simulink model "model_quad_nl_mpc_nl"  (R2021b)
settings: Solver=FixedStepAuto  StartTime=0.0  StopTime=10  FixedStep=.01  MaxStep=.1  MinStep=.005  RelTol=1e-3
values from neighbouring files (symbols this model uses):
  Abody = pi*Rbody^2    (= 0.0314159265359)    [model_quad_init.m]    (also in nlStateFcn.m = 0.0314)
  CDbody = 0.75    [model_quad_init.m]    (also in nlStateFcn.m)
  CT = 0.0248    [model_quad_init.m]
  g = 9.81    [model_quad_init.m]    (also in nlStateFcn.m; nlStateFcnTest.m; start_drone.m)
  i0 = 0    [model_quad_init.m]    (also in nlStateFcn.m)
  Ibbperp = .00942    (= 0.00942)    [model_quad_init.m]    (also in nlStateFcn.m; nlStateFcnTest.m)
  Ibbxx = Ibbperp    (= 0.00942)    [model_quad_init.m]    (also in nlStateFcn.m; nlStateFcnTest.m)
  Ibbxz = 0    [model_quad_init.m]    (also in nlStateFcn.m; nlStateFcnTest.m)
  Ibbyy = Ibbperp    (= 0.00942)    [model_quad_init.m]    (also in nlStateFcn.m; nlStateFcnTest.m)
  Ibbzz = .01867    (= 0.01867)    [model_quad_init.m]    (also in nlStateFcn.m; nlStateFcnTest.m)
  Irrperp = Irrpolar/2    (= 0.0001113)    [model_quad_init.m]    (also in nlStateFcn.m; nlStateFcnTest.m)
  Irrpolar = .0002226    (= 0.0002226)    [model_quad_init.m]
  Kv = 130    [model_quad_init.m]    (also in nlStateFcn.m)
  mb = mb/m_tot    (= 0.760306807287)    [model_quad_init.m]    (also in nlStateFcn.m; nlStateFcnTest.m)
  mr = mr/m_tot    (= 0.0599232981783)    [model_quad_init.m]    (also in nlStateFcn.m; nlStateFcnTest.m)
  R_arms = .45/2    (= 0.225)    [model_quad_init.m]    (also in nlStateFcn.m; nlStateFcnTest.m)
  R_rotor = .125    (= 0.125)    [model_quad_init.m]    (also in nlStateFcn.m)
  rho = 1.225    [model_quad_init.m]    (also in nlStateFcn.m)
  rotorAero = load('loopQuadBET_fromTheBook.mat','C_T','C_H','C_M','C_Q','mu_z_loops','mu_x_loops')    [model_quad_init.m]    (also in nlStateFcn.m)
  Rwinding = 0.56    [model_quad_init.m]
  spin_dir = [1 -1 1 -1]    [model_quad_init.m]    (also in nlStateFcn.m = [1,-1,1,-1])
  Vmax = 4*3.7    (= 14.8)    [model_quad_init.m]
  z_rotors = 0    [model_quad_init.m]    (also in nlStateFcn.m; nlStateFcnTest.m)
undefined symbols (not defined in the file or in its folder): R_RB
libraries: dspmathops x1, mpclib x1
(part 2 of 2)

== matlab function model_quad_nl_mpc_nl/NL Drone Model/Aerodynamics/rotor aerodynamics2/MATLAB Function ==
  data: Omega1 input; Omega2 input; Omega3 input; Omega4 input; R input; phi input; psi input; theta input; u input; mu output; v input; w input; w_xE input; w_yE input; w_zE input
function mu = ODE_quad_advanceratios(Omega1,Omega2,Omega3,Omega4,R,phi,psi,theta,u,v,w,w_xE,w_yE,w_zE)
%ODE_QUAD_ADVANCERATIOS
%    MU = ODE_QUAD_ADVANCERATIOS(OMEGA1,OMEGA2,OMEGA3,OMEGA4,R,PHI,PSI,THETA,U,V,W,W_XE,W_YE,W_ZE)

%    This function was generated by the Symbolic Math Toolbox version 8.5.
%    12-Apr-2021 01:36:09

t2 = cos(phi);
t3 = cos(psi);
t4 = cos(theta);
t5 = sin(phi);
t6 = sin(psi);
t7 = sin(theta);
t8 = 1.0./Omega1;
t9 = 1.0./Omega2;
t10 = 1.0./Omega3;
t11 = 1.0./Omega4;
t12 = 1.0./R;
t13 = t7.*w_zE;
t14 = t2.*t3;
t15 = t2.*t6;
t16 = t3.*t5;
t17 = t5.*t6;
t18 = t2.*t4.*w_zE;
t19 = t3.*t4.*w_xE;
t20 = t4.*t5.*w_zE;
t21 = t4.*t6.*w_yE;
t22 = t7.*t17;
t23 = t7.*t14;
t24 = t7.*t15;
t25 = t7.*t16;
t26 = -t18;
t27 = -t19;
t28 = -t20;
t29 = -t21;
t30 = -t24;
t31 = -t25;
t32 = t14+t22;
t33 = t17+t23;
t42 = t13+t27+t29+u;
t34 = t33.*w_xE;
t35 = t32.*w_yE;
t36 = t15+t31;
t37 = t16+t30;
t43 = t42.^2;
t38 = t36.*w_xE;
t39 = -t34;
t40 = t37.*w_yE;
t41 = -t35;
t44 = t28+t38+t41+v;
t45 = t26+t39+t40+w;
t46 = (t20+t35-t38-v).^2;
t47 = t43+t46;
t48 = 1.0./sqrt(t47);
t49 = t43.*t48;
t50 = t46.*t48;
t51 = t49+t50;
mu = [t8.*t12.*(t18+t34-t40-w);-t8.*t12.*t51;t9.*t12.*(t18+t34-t40-w);-t9.*t12.*t51;t10.*t12.*(t18+t34-t40-w);-t10.*t12.*t51;t11.*t12.*(t18+t34-t40-w);-t11.*t12.*t51];

== matlab function model_quad_nl_mpc_nl/NL Drone Model/Aerodynamics/rotor aerodynamics2/MATLAB Function1 ==
  data: CH1 input; CH2 input; CH3 input; CH4 input; CM1 input; FR output; CM2 input; CM3 input; CM4 input; CQ1 input; CQ2 input; CQ3 input; CQ4 input; CT1 input; CT2 input; CT3 input; CT4 input; Omega1 input; Omega2 input; Omega3 input; Omega4 input; R input; phi input; theta input; psi input; rho input; u input; v input; w_xE input; w_yE input; w_zE input
function FR = ODE_quad_rotorforces(CH1,CH2,CH3,CH4,CM1,CM2,CM3,CM4,CQ1,CQ2,CQ3,CQ4,CT1,CT2,CT3,CT4,Omega1,Omega2,Omega3,Omega4,R,phi,theta,psi,rho,u,v,w_xE,w_yE,w_zE)
%ODE_QUAD_ROTORFORCES
%    FR = ODE_QUAD_ROTORFORCES(CH1,CH2,CH3,CH4,CM1,CM2,CM3,CM4,CQ1,CQ2,CQ3,CQ4,CT1,CT2,CT3,CT4,OMEGA1,OMEGA2,OMEGA3,OMEGA4,R,PHI,PSI,RHO,THETA,U,V,W_XE,W_YE,W_ZE)

%    This function was generated by the Symbolic Math Toolbox version 8.5.
%    12-Apr-2021 00:26:00

t2 = cos(phi);
t3 = cos(psi);
t4 = cos(theta);
t5 = sin(phi);
t6 = sin(psi);
t7 = sin(theta);
t8 = Omega1.^2;
t9 = Omega2.^2;
t10 = Omega3.^2;
t11 = Omega4.^2;
t12 = R.^4;
t13 = R.^5;
t14 = t7.*w_zE;
t15 = t2.*t3;
t16 = t2.*t6;
t17 = t3.*t4.*w_xE;
t18 = t4.*t5.*w_zE;
t19 = t4.*t6.*w_yE;
t20 = t5.*t6.*t7;
t21 = t3.*t5.*t7;
t22 = -t17;
t23 = -t18;
t24 = -t19;
t25 = -t21;
t26 = t15+t20;
t27 = t26.*w_yE;
t28 = t16+t25;
t31 = t14+t22+t24+u;
t29 = t28.*w_xE;
t30 = -t27;
t32 = t31.^2;
t33 = t23+t29+t30+v;
t34 = (t18+t27-t29-v).^2;
t35 = t32+t34;
t36 = 1.0./sqrt(t35);
FR = [CH1.*rho.*t8.*t12.*t31.*t36.*pi.*(-1.0./2.0);CH2.*rho.*t9.*t12.*t31.*t36.*pi.*(-1.0./2.0);CH3.*rho.*t10.*t12.*t31.*t36.*pi.*(-1.0./2.0);CH4.*rho.*t11.*t12.*t31.*t36.*pi.*(-1.0./2.0);CH1.*rho.*t8.*t12.*t36.*pi.*(t18+t27-t29-v).*(-1.0./2.0);CH2.*rho.*t9.*t12.*t36.*pi.*(t18+t27-t29-v).*(-1.0./2.0);CH3.*rho.*t10.*t12.*t36.*pi.*(t18+t27-t29-v).*(-1.0./2.0);CH4.*rho.*t11.*t12.*t36.*pi.*(t18+t27-t29-v).*(-1.0./2.0);(CT1.*rho.*t8.*t12.*pi)./2.0;(CT2.*rho.*t9.*t12.*pi)./2.0;(CT3.*rho.*t10.*t12.*pi)./2.0;(CT4.*rho.*t11.*t12.*pi)./2.0;(CM1.*rho.*t8.*t13.*t31.*t36.*pi)./2.0;CM2.*rho.*t9.*t13.*t31.*t36.*pi.*(-1.0./2.0);(CM3.*rho.*t10.*t13.*t31.*t36.*pi)./2.0;CM4.*rho.*t11.*t13.*t31.*t36.*pi.*(-1.0./2.0);CM1.*rho.*t8.*t13.*t36.*pi.*(t18+t27-t29-v).*(-1.0./2.0);(CM2.*rho.*t9.*t13.*t36.*pi.*(t18+t27-t29-v))./2.0;CM3.*rho.*t10.*t13.*t36.*pi.*(t18+t27-t29-v).*(-1.0./2.0);(CM4.*rho.*t11.*t13.*t36.*pi.*(t18+t27-t29-v))./2.0;(CQ1.*rho.*t8.*t13.*pi)./2.0;(CQ2.*rho.*t9.*t13.*pi)./2.0;(CQ3.*rho.*t10.*t13.*pi)./2.0;(CQ4.*rho.*t11.*t13.*pi)./2.0];

== matlab function model_quad_nl_mpc_nl/NL Drone Model/Aerodynamics/rotor aerodynamics2/nozero2 ==
  data: vB input; wE2 output; wE input
function wE2 = fcn(vB,wE)

if norm([vB(:);wE(:)])==0,
    wE2=[eps;0;0];
else
    wE2=wE;
end

== matlab function model_quad_nl_mpc_nl/NL Drone Model/Flight Dynamics/DCM/MATLAB Function ==
  data: phi input; DCM output; theta input; psi input
function DCM = dcm_numeric(phi,theta,psi)
%DCM_NUMERIC
%    DCM = DCM_NUMERIC(PHI,THETA,PSI)

%    This function was generated by the Symbolic Math Toolbox version 8.5.
%    19-Oct-2020 17:32:56

t2 = cos(phi);
t3 = cos(psi);
t4 = cos(theta);
t5 = sin(phi);
t6 = sin(psi);
t7 = sin(theta);
DCM = reshape([t3.*t4,t4.*t6,-t7,-t2.*t6+t3.*t5.*t7,t2.*t3+t5.*t6.*t7,t4.*t5,t5.*t6+t2.*t3.*t7,-t3.*t5+t2.*t6.*t7,t2.*t4],[3,3]);

== matlab function model_quad_nl_mpc_nl/NL Drone Model/Flight Dynamics/ODE_Quadcopter1 ==
  data: t input; u input; out1 output; v input; w input; p input; q input; r input; x input; y input; z input; phi input; theta input; psi input; dalpha1 input; dalpha2 input; dalpha3 input; dalpha4 input; M1 input; M2 input; M3 input; M4 input; T1 input; T2 input; T3 input; T4 input; H1 input; H2 input; H3 input; H4 input; Y1 input; Y2 input; Y3 input; Y4 input; Q1 input; Q2 input; Q3 input; Q4 input; Mx1 input; Mx2 input; Mx3 input; Mx4 input; My1 input; My2 input; My3 input; My4 input; XB input; YB input; ZB input; LB input; MB input; NB input; mb input; mr input; Ibbxx input; Ibbyy input; Ibbzz input; Ibbxz input; Ibbperp input; Irrpolar input; Irrperp input; R_arms input; z_rotors input; g input
function out1 = ODE_quad(t,u,v,w,p,q,r,x,y,z,phi,theta,psi,dalpha1,dalpha2,dalpha3,dalpha4,M1,M2,M3,M4,T1,T2,T3,T4,H1,H2,H3,H4,Y1,Y2,Y3,Y4,Q1,Q2,Q3,Q4,Mx1,Mx2,Mx3,Mx4,My1,My2,My3,My4,XB,YB,ZB,LB,MB,NB,mb,mr,Ibbxx,Ibbyy,Ibbzz,Ibbxz,Ibbperp,Irrpolar,Irrperp,R_arms,z_rotors,g)
%ODE_QUAD
%    OUT1 = ODE_QUAD(T,U,V,W,P,Q,R,X,Y,Z,PHI,THETA,PSI,DALPHA1,DALPHA2,DALPHA3,DALPHA4,M1,M2,M3,M4,T1,T2,T3,T4,H1,H2,H3,H4,Y1,Y2,Y3,Y4,Q1,Q2,Q3,Q4,MX1,MX2,MX3,MX4,MY1,MY2,MY3,MY4,XB,YB,ZB,LB,MB,NB,MB,MR,IBBXX,IBBYY,IBBZZ,IBBXZ,IBBPERP,IRRPOLAR,IRRPERP,R_ARMS,Z_ROTORS,G)

%    This function was generated by the Symbolic Math Toolbox version 8.5.
%    03-Jan-2021 19:34:45

t2 = cos(phi);
t3 = cos(psi);
t4 = cos(theta);
t5 = sin(phi);
t6 = sin(psi);
t7 = sin(theta);
t8 = Irrperp.*4.0;
t9 = R_arms.^2;
t10 = mr.*4.0;
t11 = 1.0./Irrpolar;
t12 = -Q1;
t13 = -Q2;
t14 = -Q3;
t15 = -Q4;
t17 = sqrt(2.0);
t16 = 1.0./t4;
t18 = mb+t10;
t19 = M1+t12;
t20 = M2+t13;
t21 = M3+t14;
t22 = M4+t15;
t23 = mr.*t9.*2.0;
t24 = t9.*t10;
t35 = (H1.*R_arms.*t17)./2.0;
t36 = (H2.*R_arms.*t17)./2.0;
t37 = (H3.*R_arms.*t17)./2.0;
t38 = (H4.*R_arms.*t17)./2.0;
t39 = (R_arms.*T1.*t17)./2.0;
t40 = (R_arms.*T2.*t17)./2.0;
t41 = (R_arms.*T3.*t17)./2.0;
t42 = (R_arms.*T4.*t17)./2.0;
t43 = (R_arms.*Y1.*t17)./2.0;
t44 = (R_arms.*Y2.*t17)./2.0;
t45 = (R_arms.*Y3.*t17)./2.0;
t46 = (R_arms.*Y4.*t17)./2.0;
t25 = Irrpolar.*t19;
t26 = Irrpolar.*t20;
t27 = Irrpolar.*t21;
t28 = Irrpolar.*t22;
t29 = Ibbzz+t24;
t30 = 1.0./t18;
t48 = Ibbperp+t8+t23;
t49 = -t36;
t50 = -t37;
t51 = -t42;
t52 = -t45;
t53 = -t46;
t31 = -t25;
t32 = -t26;
t33 = -t27;
t34 = -t28;
t47 = 1.0./t29;
t54 = 1.0./t48;
t55 = NB+Q2+Q4+t12+t14+t35+t38+t43+t44+t49+t50+t52+t53;
t56 = Irrpolar.*t55;
t57 = -t56;
out1 = [-q.*w+r.*v-t30.*(H1+H2+H3+H4-XB+g.*t7.*t18);t30.*(Y1+Y2+Y3+Y4+YB+g.*t4.*t5.*t18)+p.*w-r.*u;-p.*v+q.*u-t30.*(T1+T2+T3+T4-ZB-g.*t2.*t4.*t18);t54.*(LB+Mx1+Mx2+Mx3+Mx4-t39+t40+t41+t51-Irrpolar.*dalpha1.*q+Irrpolar.*dalpha2.*q-Irrpolar.*dalpha3.*q+Irrpolar.*dalpha4.*q-Ibbzz.*q.*r+Ibbperp.*q.*r-Irrpolar.*q.*r.*4.0+q.*r.*t8-mr.*q.*r.*t9.*2.0);t54.*(MB+My1+My2+My3+My4+t39+t40-t41+t51+Irrpolar.*dalpha1.*p-Irrpolar.*dalpha2.*p+Irrpolar.*dalpha3.*p-Irrpolar.*dalpha4.*p+Ibbzz.*p.*r-Ibbperp.*p.*r-Irrperp.*p.*r.*4.0+Irrpolar.*p.*r.*4.0+p.*r.*t23);t47.*(-M1+M2-M3+M4+NB+t35+t38+t43+t44+t49+t50+t52+t53);t3.*t4.*u-t2.*t6.*v+t5.*t6.*w+t3.*t5.*t7.*v+t2.*t3.*t7.*w;t4.*t6.*u+t2.*t3.*v-t3.*t5.*w+t5.*t6.*t7.*v+t2.*t6.*t7.*w;-t7.*u+t4.*t5.*v+t2.*t4.*w;t16.*(p.*t4+q.*t5.*t7+r.*t2.*t7);q.*t2-r.*t5;t16.*(q.*t5+r.*t2);t11.*t47.*(t25+t27+t32+t34+t57+Ibbzz.*t19+t19.*t24);t11.*t47.*(t26+t28+t31+t33+t56+Ibbzz.*t20+t20.*t24);t11.*t47.*(t25+t27+t32+t34+t57+Ibbzz.*t21+t21.*t24);t11.*t47.*(t26+t28+t31+t33+t56+Ibbzz.*t22+t22.*t24)];

== matlab function model_quad_nl_mpc_nl/NL Drone Model/Motors/motor_function/MATLAB Function ==
  data: K_v input; M output; Omega1 input; Omega2 input; Omega3 input; Omega4 input; R_winding input; V1 input; V2 input; V3 input; V4 input
function M = ODE_quad_motors(K_v,Omega1,Omega2,Omega3,Omega4,R_winding,V1,V2,V3,V4)
%ODE_QUAD_MOTORS
%    M = ODE_QUAD_MOTORS(K_V,OMEGA1,OMEGA2,OMEGA3,OMEGA4,R_WINDING,V1,V2,V3,V4)

%    This function was generated by the Symbolic Math Toolbox version 8.5.
%    12-Apr-2021 01:36:03

t2 = 1.0./K_v;
t3 = 1.0./R_winding;
M = [t2.*t3.*(V1-Omega1.*t2);t2.*t3.*(V2-Omega2.*t2);t2.*t3.*(V3-Omega3.*t2);t2.*t3.*(V4-Omega4.*t2)];

== matlab function model_quad_nl_mpc_nl/NL Drone Model/Aerodynamics/body aerodynamics1/MATLAB Function ==
  data: A_body input; C_Dbody input; phi input; psi input; rho input; theta input; u input; FB output; v input; w input; w_xE input; w_yE input; w_zE input
function FB = ODE_quad_bodyforces(A_body,C_Dbody,phi,psi,rho,theta,u,v,w,w_xE,w_yE,w_zE)
%ODE_QUAD_BODYFORCES
%    FB = ODE_QUAD_BODYFORCES(A_BODY,C_DBODY,PHI,PSI,RHO,THETA,U,V,W,W_XE,W_YE,W_ZE)

%    This function was generated by the Symbolic Math Toolbox version 8.5.
%    12-Apr-2021 00:25:58

t2 = cos(phi);
t3 = cos(psi);
t4 = cos(theta);
t5 = sin(phi);
t6 = sin(psi);
t7 = sin(theta);
t8 = t7.*w_zE;
t9 = t2.*t3;
t10 = t2.*t6;
t11 = t3.*t5;
t12 = t5.*t6;
t13 = t2.*t4.*w_zE;
t14 = t3.*t4.*w_xE;
t15 = t4.*t5.*w_zE;
t16 = t4.*t6.*w_yE;
t17 = t7.*t12;
t18 = t7.*t9;
t19 = t7.*t10;
t20 = t7.*t11;
t21 = -t13;
t22 = -t14;
t23 = -t15;
t24 = -t16;
t25 = -t19;
t26 = -t20;
t27 = t9+t17;
t28 = t12+t18;
t37 = t8+t22+t24+u;
t29 = t28.*w_xE;
t30 = t27.*w_yE;
t31 = t10+t26;
t32 = t11+t25;
t38 = abs(t37);
t33 = t31.*w_xE;
t34 = -t29;
t35 = t32.*w_yE;
t36 = -t30;
t39 = t38.^2;
t40 = t23+t33+t36+v;
t41 = t21+t34+t35+w;
t42 = abs(t41);
t43 = abs(t40);
t44 = t42.^2;
t45 = t43.^2;
t46 = t39+t44+t45;
t47 = sqrt(t46);
FB = [A_body.*C_Dbody.*rho.*t37.*t47.*(-1.0./2.0);(A_body.*C_Dbody.*rho.*t47.*(t15+t30-t33-v))./2.0;(A_body.*C_Dbody.*rho.*t47.*(t13+t29-t35-w))./2.0;0.0;0.0;0.0];

== matlab function model_quad_nl_mpc_nl/NL Drone Model/Aerodynamics/rotor aerodynamics/rotor_aero_lookup2/Subsystem/MATLAB Function ==
  data: vB input; R_RW output; R_BR input; vW output
function [R_RW,vW] = toXZplane(vB,R_BR)
% vB is vehicle velocity vector in body coords (IAS - i.e. relative to
% local air; wind must be inverted)
% R_BRa is rotation matrix from body frame to rotor frame (z along shaft, x
% usually forwards)
% R_RW is rotation matrix from rotor frame to wind frame (z aligned with
% shaft, wind aligned with xz plane)
% vW is the 3 element wind vector transformed by R_RW.' to lie in the "wind
% frame" where only the 1st and 3rd elements can be nonzero.

% define output sizes
R_RW = zeros(3,3);
vW   = zeros(3,1);

% convert vehicle velocity in body frame to relative wind velocity in rotor frame
vR = -R_BR.'*vB(:);

% determine transform to align rotor XZ plane with relative wind (R is
% nominal rotor frame, W is rotated about z to align wind in XZ plane)
if vR(1)==0 && vR(2)==0, % wind is zero or aligned with Z axis
    R_RW = eye(3);
else
    h = (vR(1)^2 + vR(2)^2)^0.5; % size of vR projected on XY plane (NB this is mu_x component)
    %a = atan2(vW(2),vW(1)) 
    c = vR(1)/h; %cos(a); 
    s = vR(2)/h; %sin(a);
    R_RW = [ c -s 0 ; s c 0 ; 0 0 1];
end

% get relative wind in XZ plane
vW = R_RW.' * vR;

== matlab function model_quad_nl_mpc_nl/NL Drone Model/Aerodynamics/rotor aerodynamics/rotor_aero_lookup2/Subsystem1/MATLAB Function ==
  data: vB input; R_RW output; R_BR input; vW output
function [R_RW,vW] = toXZplane(vB,R_BR)
% vB is vehicle velocity vector in body coords (IAS - i.e. relative to
% local air; wind must be inverted)
% R_BRa is rotation matrix from body frame to rotor frame (z along shaft, x
% usually forwards)
% R_RW is rotation matrix from rotor frame to wind frame (z aligned with
% shaft, wind aligned with xz plane)
% vW is the 3 element wind vector transformed by R_RW.' to lie in the "wind
% frame" where only the 1st and 3rd elements can be nonzero.

% define output sizes
R_RW = zeros(3,3);
vW   = zeros(3,1);

% convert vehicle velocity in body frame to relative wind velocity in rotor frame
vR = -R_BR.'*vB(:);

% determine transform to align rotor XZ plane with relative wind (R is
% nominal rotor frame, W is rotated about z to align wind in XZ plane)
if vR(1)==0 && vR(2)==0, % wind is zero or aligned with Z axis
    R_RW = eye(3);
else
    h = (vR(1)^2 + vR(2)^2)^0.5; % size of vR projected on XY plane (NB this is mu_x component)
    %a = atan2(vW(2),vW(1)) 
    c = vR(1)/h; %cos(a); 
    s = vR(2)/h; %sin(a);
    R_RW = [ c -s 0 ; s c 0 ; 0 0 1];
end

% get relative wind in XZ plane
vW = R_RW.' * vR;
